simulink model "PLL"  (R2020a)
settings: Solver=VariableStepAuto  StartTime=0.0  StopTime=0.5  RelTol=1e-3
libraries: powerlib_meascontrol x3
settings Model: Creator=Naeem Mohammad  LastModifiedBy=Naeem Mohammad

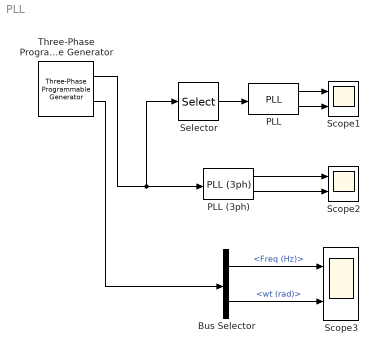
== system PLL ==
  Bus Selector : BusSelector  OutputSignals=Freq (Hz),wt (rad)
  PLL : powerlib_meascontrol/PLL/PLL  Fmin=45  Par_Init=[0, 60]  ParK=[180, 3200, 1]  TcD=1e-3  MaxRateChangeFreq=12  FilterCutOffFreq=25  Ts=0  AGC=on
      settings: SourceProductBaseCode=PS
  PLL (3ph) : powerlib_meascontrol/PLL/PLL (3ph)  Fmin=45  Par_Init=[0, 60]  ParK=[180, 3200, 1]  TcD=1e-4  MaxRateChangeFreq=12  FilterCutOffFreq=25  Ts=0  AGC=on
  Scope1 : Scope  NumInputPorts=2
  Scope2 : Scope  NumInputPorts=2
  Scope3 : Scope  NumInputPorts=2
  Selector : Selector  InputPortWidth=3  IndexOptions=Index vector (dialog)  Indices=1  OutputSizes=1
  Three-Phase Programmable Generator : powerlib_meascontrol/Pulse & Signal Generators/Three-Phase Programmable Generator  Par_Vps=[100, 0, 60]  VariationEntity=Frequency  VariationType=Step  VariationStep=0.5  VariationRate=10  VariationMag=0.3  VariationFreq=2  Par_Timing_Variation="[0.2  1.2]"  SinglePhase=on  Yampli=[1 0.2 1.2 1.0]  Xtime=[0 0.1 0.15 0.2]  HarmonicGeneration=off  Par_HarmoA="[3  5  -25 0]"  Par_HarmoB="[5  10  35  2]"  Par_Timing_Harmo="[ 0.05  99]"  Ts=0
      settings: SourceProductBaseCode=PS
  wires:
  PLL/1 -> Scope1/1
  Three-Phase Programmable Generator/1 -> Selector/1, PLL (3ph)/1
  PLL (3ph)/1 -> Scope2/1
  PLL (3ph)/2 -> Scope2/2
  Three-Phase Programmable Generator/2 -> Bus Selector/1
  PLL/2 -> Scope1/2
  Selector/1 -> PLL/1
  Bus Selector/1 -> Scope3/1  "<Freq (Hz)>"
  Bus Selector/2 -> Scope3/2  "<wt (rad)>"
